simulink model "matusek_misik"  (R2016b)
settings: Solver=VariableStepAuto  StartTime=0.0  StopTime=5000  RelTol=1e-3
values from neighbouring files (symbols this model uses):
  F_den = double(coeffs(F_d))    [matausek_misic.m]
  F_num = double(coeffs(F_n))    [matausek_misic.m]
  Ki = -0.075    [defineparams.m]    (also in smithpredictor_1.m)
  Km = 4    [defineparams.m]    (also in smithpredictor_1.m)
  Kp = -0.1    [matausek_misic.m]
  Kr = -0.1    [matausek_misic.m]
  Tdi = 25    [defineparams.m]    (also in smithpredictor_1.m)
  Tdm = 15    [defineparams.m]    (also in smithpredictor_1.m)
  Ti = 140    [defineparams.m]    (also in smithpredictor_1.m)
  Tm = 50    [defineparams.m]    (also in smithpredictor_1.m)
settings Model: Creator=Matt Cordoba  LastModifiedBy=Matt Cordoba

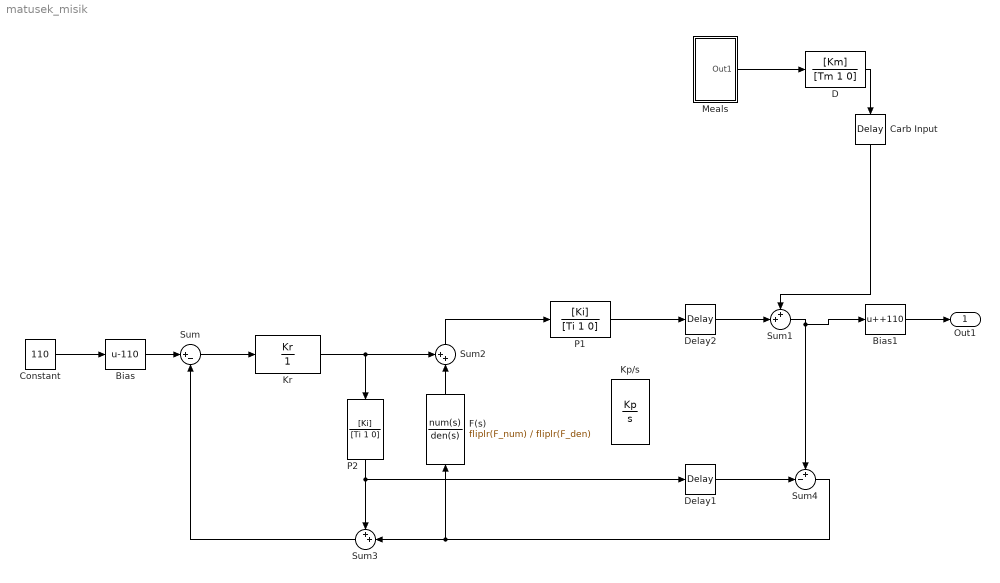
== system matusek_misik ==
  " Kr" : TransferFcn  Numerator=Kr  Denominator=1
  Bias : Bias  Bias=-110
  Bias1 : Bias  Bias=+110
  Carb Input : TransportDelay  DelayTime=Tdm
  Constant : Constant  Value=110
  D : TransferFcn  Numerator=[Km]  Denominator=[Tm 1 0]
  Delay1 : TransportDelay  DelayTime=Tdi
  Delay2 : TransportDelay  DelayTime=Tdi
  "F(s) " : TransferFcn  Numerator=fliplr(F_num)  Denominator=fliplr(F_den)
  Kp/s : TransferFcn  Numerator=Kp  Denominator=[1 0]
  Meals : Subsystem
  P1 : TransferFcn  Numerator=[Ki]  Denominator=[Ti 1 0]
  P2 : TransferFcn  Numerator=[Ki]  Denominator=[Ti 1 0]
  Sum : Sum  Inputs=|+-
  Sum1 : Sum  Inputs=++|
  Sum2 : Sum  Inputs=++|
  Sum3 : Sum  Inputs=++|
  Sum4 : Sum  Inputs=+-|
  Out1 : Outport
  wires:
  Sum3/1 -> Sum/2
  Constant/1 -> Bias/1
  Bias/1 -> Sum/1
  Sum/1 -> " Kr"/1
  " Kr"/1 -> P2/1, Sum2/1
  P2/1 -> Delay1/1, Sum3/1
  P1/1 -> Delay2/1
  Delay2/1 -> Sum1/2
  Sum2/1 -> P1/1
  "F(s) "/1 -> Sum2/2
  Delay1/1 -> Sum4/2
  Sum4/1 -> "F(s) "/1, Sum3/2
  D/1 -> Carb Input/1
  Meals/1(Out1) -> D/1
  Carb Input/1 -> Sum1/1
  Sum1/1 -> Bias1/1, Sum4/1
  Bias1/1 -> Out1/1

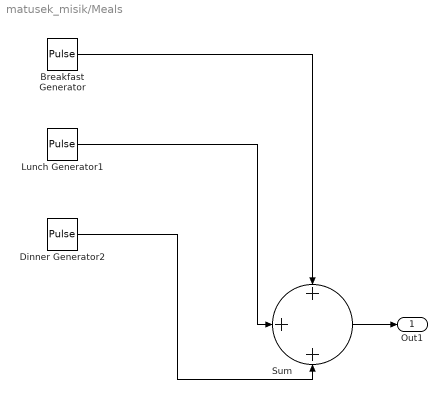
== system matusek_misik/Meals ==
  Breakfast Generator : DiscretePulseGenerator  Amplitude=25/10  Period=1440  PulseWidth=10  PhaseDelay=420
  Dinner Generator2 : DiscretePulseGenerator  Amplitude=3  Period=1440  PulseWidth=20  PhaseDelay=1080
  Lunch Generator1 : DiscretePulseGenerator  Amplitude=40/15  Period=1440  PulseWidth=15  PhaseDelay=780
  Sum : Sum  Inputs=+++
  Out1 : Outport
  wires:
  Breakfast Generator/1 -> Sum/1
  Lunch Generator1/1 -> Sum/2
  Dinner Generator2/1 -> Sum/3
  Sum/1 -> Out1/1
